simulink model "Bixler_w_autopilot_sepTaskRate"  (R2018b)
settings: Solver=FixedStepAuto  StartTime=0.0  StopTime=inf  RelTol=1e-3  EnableMultiTasking=on
undefined symbols (not defined in the file or in its folder): dev, Main, pwm_output0
libraries: simulink x5, px4uORBlib x5, aerolibutil x4, px4lib x2, px4Sensorslib x2, vrlib x1, sharedtransform x1
(part 1 of 2)
settings Model: xpc_rtwmakecfg_data=_xpcnblib_  SimulationMode=external  ExtModeTrigDuration=10  Creator=Robert  LastModifiedBy=Robert
settings SolverCC: PositivePriorityOrder=on
settings DataIOCC: SaveState=on
settings OptimizationCC: DefaultUnderspecifiedDataType=single  EnhancedBackFolding=on  PassReuseOutputArgsAs=Individual arguments  MaxStackSize=64  OptimizeBlockOrder=speed  DifferentSizesBufferReuse=on  OptimizationCustomize=off
settings DebuggingCC: ParameterTunabilityLossMsg=error
settings HardwareCC: ProdBitPerPointer=32  ProdBitPerSizeT=32  ProdBitPerPtrDiffT=32  ProdLargestAtomicInteger=Long  ProdLargestAtomicFloat=Double  ProdWordSize=32  ProdLongLongMode=on  ProdHWDeviceType=ARM Compatible->ARM Cortex
settings SFSimCC: MATLABDynamicMemAlloc=off
settings RTWCC: SystemTargetFile=ert.tlc  HardwareBoard=PX4 Pixhawk 1  TLCOptions="-aInlineSetEventsForThisBaseRateFcn=TLC_FALSE -aSuppressMultiTaskScheduler=TLC_FALSE  -aRateBasedStepFcn=0"  TemplateMakefile=ert_default_tmf  GenerateReport=on  Toolchain=GNU Tools for PX4 Autopilots  IncludeHyperlinkInReport=on  LaunchReport=on  TargetLang=C++  GenerateTraceInfo=on  GenerateTraceReport=on  GenerateTraceReportSl=on  GenerateTraceReportSf=on  GenerateTraceReportEml=on
settings CodeAppCC: ForceParamTrailComments=on  IgnoreCustomStorageClasses=off  OperatorAnnotations=on  SimulinkDataObjDesc=on  SFDataObjDesc=on  InsertBlockDesc=on
settings ERTTargetCC: ExtMode=on  ExtModeMexArgs='127.0.0.1' 1 17725

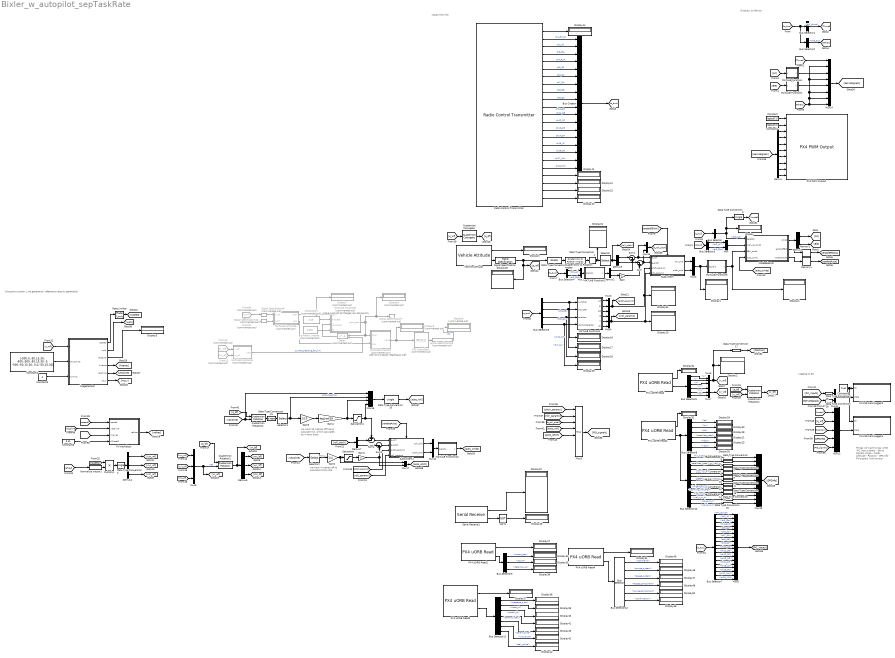
== system Bixler_w_autopilot_sepTaskRate ==
  note: Logging to SD
  note: Inputs from RC
  note: Outputs, to Servos
  note: Things we want to log:
      |
      | uint8
      | -RC input signals
      | - Servo Signals
      |
      | single
      | - Mode
      | - Attitude
      | - Position
      | - GPS info
      | - Pid signals (with errors)
  note: we want 4 metres off
      | to saturate climb rate
  note: Waypoint system,
      | Line generation,
      | reference velocity generation
  note: make sure not to change yaw too quickly
  note: Use roll to adjust heading as well
  note: we want 10 metres off
      | line to saturate roll, which
      | saturates as in next block
  Bus Creator : BusCreator  Inputs=18
  Bus Selector : BusSelector  OutputSignals=ch9_SC
  Bus Selector1 : BusSelector  OutputSignals=ch1_thrust
  Bus Selector10 : BusSelector  OutputSignals=fix_type,satellites_used,lat,lon,alt,hdop,vdop,noise_per_ms,jamming_indicator,vel_m_s,vel_n_m_s,vel_e_m_s,vel_d_m_s
  Bus Selector11 : BusSelector  OutputSignals=message_type,node_id,param_id,param_index,param_type,int_value,real_value
  Bus Selector12 : BusSelector  OutputSignals=command,source_system,target_system,target_component,source_component,confirmation
  Bus Selector2 : BusSelector  OutputSignals=ch6_S2
  Bus Selector3 : BusSelector  OutputSignals=ch2_Ail,ch3_Ele
  Bus Selector4 : BusSelector  OutputSignals=ch2_Ail,ch3_Ele
  Bus Selector5 : BusSelector  OutputSignals=ch8_SB,ch5_S1,ch12_SF,ch7_SA
  Bus Selector6 : BusSelector  OutputSignals=x,y,z,vx,vy,vz
  Bus Selector7 : BusSelector  OutputSignals=ch1_thrust,ch2_Ail,ch3_Ele,ch4_Rud,ch5_S1,ch6_S2,ch7_SA,ch8_SB,ch9_SC,ch10_SD,ch11_SE,ch12_SF,ch13_SG,ch14_SH,ch15_LS,ch16_RS,ch17_MAX,ch18_MIN
  Bus Selector8 : BusSelector  OutputSignals=lat,lon,alt,satellites_used,hdop,vdop
  Bus Selector9 : BusSelector  OutputSignals=current_seq,count,dataman_id
  Constant : Constant  Value=logical(1)
  Constant1 : Constant  Value=logical(0)
  Constant11 : Constant  Commented=on  Value=0.15  OutDataTypeStr=single  SampleTime=1/250
  Constant2 : Constant  Value=[-500,0,-50,15,30; -500,-500,-50,15,30; 0, -500,-50,15,30; 0,0,-50,15,30]  OutDataTypeStr=single
  Constant3 : Constant  Value=4  OutDataTypeStr=single
  Constant5 : Constant  Value=0.11  OutDataTypeStr=single  SampleTime=-1
  Constant8 : Constant  Value=true  OutDataTypeStr=boolean  SampleTime=0.004
  Data Type Conversion : DataTypeConversion  OutDataTypeStr=double
  Data Type Conversion{1..17,20..21} (19 alike) : DataTypeConversion  OutDataTypeStr=single
  Data Type Conversion18 : DataTypeConversion  OutDataTypeStr=uint16
  Data Type Conversion19 : DataTypeConversion  OutDataTypeStr=uint16
  Delay : Delay  Commented=on  DelayLength=1  InitialConditionSource=Input port
      settings: InputPortMap=u0,p4
  Demux : Demux  Outputs=8
  Demux{1..3,7} (4 alike) : Demux  Outputs=2
  Demux4 : Demux  Outputs=3
  Demux5 : Demux  Outputs=3
  Display{,1..5,10..51} (48 alike) : Display
  Display{6..9} (4 alike) : Display  Commented=on
  FlyVecAdjust : MATLAB Function  TreatAsAtomicUnit=on
  From12 : From  Commented=on  GotoTag=v_wf
  From13 : From  Commented=on  GotoTag=vr_wf
  From56 : From  Commented=on  GotoTag=vr_wf
  From57 : From  Commented=on  GotoTag=v_wf
  Gain : Gain  Gain=-1
  Gain1 : Gain  Gain=-1
  Gain2 : Gain  Gain=1/4
  Gain3 : Gain  Gain=1/10
  Gain4 : Gain  Gain=deg2rad(30)
  MATLAB Function : MATLAB Function  TreatAsAtomicUnit=on
  MATLAB Function1 : MATLAB Function  TreatAsAtomicUnit=on
  MATLAB Function10 : MATLAB Function  TreatAsAtomicUnit=on
  MATLAB Function2 : MATLAB Function  TreatAsAtomicUnit=on
  MATLAB Function3 : MATLAB Function  TreatAsAtomicUnit=on
  MATLAB Function4 : MATLAB Function  TreatAsAtomicUnit=on
  MATLAB Function5 : MATLAB Function  Commented=on  TreatAsAtomicUnit=on
  MATLAB Function6 : MATLAB Function  Commented=on  TreatAsAtomicUnit=on
  MATLAB Function7 : MATLAB Function  Commented=on  TreatAsAtomicUnit=on
  MATLAB Function8 : MATLAB Function  Commented=on  TreatAsAtomicUnit=on
  Memory1 : Memory  InheritSampleTime=on
  Memory2 : Memory  InheritSampleTime=on
  ModeSelector : MATLAB Function  TreatAsAtomicUnit=on
  Multiply1 : Product
  Mux{,1..2,10..11,15,17} (7 alike) : Mux  Inputs=2
  Mux12 : Mux  Inputs=5
  Mux13 : Mux  Inputs=13
  Mux14 : Mux  Inputs=8
  Mux16 : Mux
  Mux{3..7} (5 alike) : Mux  Inputs=3
  Mux8 : Mux  Inputs=18
  Mux9 : Mux  Inputs=8
  NOT1 : Logic  Operator=NOT  IconShape=distinctive  AllPortsSameDT=off  OutDataTypeStr=boolean
  Normalize Vector1 : vrlib/Utilities/Normalize Vector  maxzero=0
      settings: SourceProductName=Simulink 3D Animation  SourceProductBaseCode=VR
  PID Controller2 : simulink/Continuous/PID Controller  Commented=on  Controller=PID  Form=Parallel  TimeDomain=Discrete-time  SampleTime=-1  IntegratorMethod=Forward Euler  FilterMethod=Forward Euler  ControllerParametersSource=internal  P=1  I=0  D=0.5*0  UseFilter=off  N=100  TunerSelectOption=Transfer Function Based (PID Tuner App)  InitialConditionSource=internal  InitialConditionForIntegrator=0  InitialConditionForFilter=0  DifferentiatorICPrevScaledInput=0  ExternalReset=none  TrackingMode=off  Kt=1  LimitOutput=on  UpperSaturationLimit=deg2rad(30)  LowerSaturationLimit=-deg2rad(30)  LinearizeAsGain=on  AntiWindupMode=clamping  Kb=1  POutMin=[]  POutMax=[]  IOutMin=[]  IOutMax=[]  DOutMin=[]  DOutMax=[]  NOutMin=[]  NOutMax=[]  SumOutMin=[]  SumOutMax=[]  SaturationOutMin=[]  SaturationOutMax=[]  PParamMin=[]  PParamMax=[]  IParamMin=[]  IParamMax=[]  DParamMin=[]  DParamMax=[]  NParamMin=[]  NParamMax=[]  KbParamMin=[]  KbParamMax=[]  KtParamMin=[]  KtParamMax=[]  KbOutMin=[]  KbOutMax=[]  KtOutMin=[]  KtOutMax=[]  IntegratorOutMin=[]  IntegratorOutMax=[]  FilterOutMin=[]  FilterOutMax=[]  SumI1OutMin=[]  SumI1OutMax=[]  SumI2OutMin=[]  SumI2OutMax=[]  SumI3OutMin=[]  SumI3OutMax=[]  SumI4OutMin=[]  SumI4OutMax=[]  SumDOutMin=[]  SumDOutMax=[]  DifferentiatorOutMin=[]  DifferentiatorOutMax=[]  FilterDiffOutCoefMin=[]  FilterDiffOutCoefMax=[]  ReciprocalOutMin=[]  ReciprocalOutMax=[]  SumDenOutMin=[]  SumDenOutMax=[]  SumNumOutMin=[]  SumNumOutMax=[]  DivideOutMin=[]  DivideOutMax=[]  IntegratorContinuousStateAttributes=''  IntegratorStateMustResolveToSignalObject=off  IntegratorRTWStateStorageClass=Auto  FilterContinuousStateAttributes=''  FilterStateMustResolveToSignalObject=off  FilterRTWStateStorageClass=Auto  ParallelPVariant=InternalParameters  IdealPVariant=Disabled  IVariant=InternalParameters  DVariant=InternalParameters  IntegratorVariant=Discrete  SatVariant=Enabled  AWVariant=DiscClampingParallel  PCopyVariant=Disabled  TRVariant=Disabled  FdbkBlocksVariant=Forward  IdealPFdbkVariant=Disabled  SatFdbkVariant=Disabled  DerivativeFilterVariant=Differentiator  NVariant=Passthrough  NCopyVariant=Disabled_SignalSpec  FilterICVariant=InternalICsDifferentiator  IntegratorICVariant=InternalICs  ExternalResetVariant=Disabled  TRSumVariant=Passthrough  SumFdbkVariant=Disabled  SumVariant=Sum_PID
  PX4 PWM Output : px4lib/PX4 PWM Output  pwmDevice=Main (/dev/pwm_output0)  pwmChannel1_=on  pwmChannel2_=on  pwmChannel3_=on  pwmChannel4_=on  pwmChannel5_=on  pwmChannel6_=on  pwmChannel7_=on  pwmChannel8_=on  forceTerminateFailsafe=off  outputErrorStatus=off
      settings: SourceProductName=Embedded Coder Support Package for PX4 Autopilots
  PX4 SD Card Logger2 : Subsystem  mask(PX4 SD Card Logger){logfile=/fs/microsd/log, logfilename=rc_and_servosignals, cacheflag=off, numRecs=250*60*60}
      mask prompts: logfile "Log Folder"; logfilename "Log File Name"; cacheflag "Cache in Memory"; numRecs "Maximum Record Count"
      mask help:
      | Log data to a specified file on the SD card
      |
      | The block accepts two inputs, enable and data. The incoming data is logged into the SD card when the enable signal is high and the number of data points logged is less than the Maximum Record Count specified.
      |
      | The specified folder should be present in the SD card for logging.
      |
      | If Cache in Memory is unchecked, the data is written to the SD card at every timestep.  If Cache in Memory is checked, data is cached in the memory and is written to SD card only when enable goes low or when the number of data points logged reaches the Maximum Record Count specified.
      mask init:
      | logname=uint8([logfile,'/',logfilename]);
      mask Help: eval('codertarget.internal.helpView(''px4'',''px4sdcardexample'')');
      mask Display:
      | fprintf([get_param(gcb,'logfile'),'/',get_param(gcb,'logfilename')])
      | port_label('input',1,'en')
      | port_label('input',2,'data')
  PX4 SD Card Logger4 : Subsystem  mask(PX4 SD Card Logger){logfile=/fs/microsd/log, logfilename=MainLog, cacheflag=off, numRecs=250*60*60}
      mask prompts: logfile "Log Folder"; logfilename "Log File Name"; cacheflag "Cache in Memory"; numRecs "Maximum Record Count"
      mask help:
      | Log data to a specified file on the SD card
      |
      | The block accepts two inputs, enable and data. The incoming data is logged into the SD card when the enable signal is high and the number of data points logged is less than the Maximum Record Count specified.
      |
      | The specified folder should be present in the SD card for logging.
      |
      | If Cache in Memory is unchecked, the data is written to the SD card at every timestep.  If Cache in Memory is checked, data is cached in the memory and is written to SD card only when enable goes low or when the number of data points logged reaches the Maximum Record Count specified.
      mask init:
      | logname=uint8([logfile,'/',logfilename]);
      mask Help: eval('codertarget.internal.helpView(''px4'',''px4sdcardexample'')');
      mask Display:
      | fprintf([get_param(gcb,'logfile'),'/',get_param(gcb,'logfilename')])
      | port_label('input',1,'en')
      | port_label('input',2,'data')
  PX4 uORB Read : px4uORBlib/PX4 uORB Read  uORBTopic=vehicle_local_position  sampleTime=0.004  BlockingMode=off  BlockTimeout=1e-3
      settings: SourceProductName=Embedded Coder Support Package for PX4 Autopilots
  PX4 uORB Read1 : px4uORBlib/PX4 uORB Read  uORBTopic=mission  sampleTime=-1  BlockingMode=off  BlockTimeout=1e-3
      settings: SourceProductName=Embedded Coder Support Package for PX4 Autopilots
  PX4 uORB Read2 : px4uORBlib/PX4 uORB Read  uORBTopic=vehicle_gps_position  sampleTime=0.004  BlockingMode=off  BlockTimeout=1e-3
      settings: SourceProductName=Embedded Coder Support Package for PX4 Autopilots
  PX4 uORB Read3 : px4uORBlib/PX4 uORB Read  uORBTopic=uavcan_parameter_request  sampleTime=-1  BlockingMode=off  BlockTimeout=1e-3
      settings: SourceProductName=Embedded Coder Support Package for PX4 Autopilots
  PX4 uORB Read4 : px4uORBlib/PX4 uORB Read  uORBTopic=vehicle_command  sampleTime=-1  BlockingMode=off  BlockTimeout=1e-3
      settings: SourceProductName=Embedded Coder Support Package for PX4 Autopilots
  Quaternion Conjugate : aerolibutil/Quaternion Conjugate
      settings: SourceProductName=Aerospace Blockset  SourceProductBaseCode=AE
  Quaternion Rotation1 : aerolibutil/Quaternion Rotation
  Quaternion Rotation2 : aerolibutil/Quaternion Rotation
  Quaternion Rotation4 : aerolibutil/Quaternion Rotation
  Quaternions to Rotation Angles : sharedtransform/Quaternions to Rotation Angles  rotationOrder=ZYX  aMode=aMode
      settings: SourceProductBaseCode=AE
  Radio Control Transmitter : px4Sensorslib/Radio Control Transmitter  channel1=on  channel2=on  channel3=on  channel4=on  channel5=on  channel6=on  channel7=on  channel8=on  channel9=on  channel10=on  channel11=on  channel12=on  channel13=on  channel14=on  channel15=on  channel16=on  channel17=on  channel18=on  channel_count=on  rssi=on  rc_input_source=on  timestamp_last_signal=on  time_stamp=off  sampleTime=1/250  BlockingMode=off  BlockTimeout=5
      settings: SourceProductName=Embedded Coder Support Package for PX4 Autopilots
  Rate Limiter : RateLimiter  SampleTimeMode=inherited  InitialCondition=0.01
  Saturation : Saturate  UpperLimit=deg2rad(15)  LowerLimit=deg2rad(-20)
  Saturation1 : Saturate  UpperLimit=deg2rad(30)  LowerLimit=deg2rad(-30)
  Selector : Selector  InputPortWidth=3  IndexOptions=Index vector (dialog)  Indices=[3 2]  OutputSizes=1
  Selector1 : Selector  InputPortWidth=3  IndexOptions=Index vector (dialog)  Indices=[2]  OutputSizes=1
  Selector2 : Selector  InputPortWidth=3  IndexOptions=Index vector (dialog)  Indices=[3]  OutputSizes=1
  Serial Receive1 : px4lib/Serial Receive  SCIModule=/dev/ttyS2  DataType=uint8  DataLength=10  OutputStatus=on  SampleTime=-1  BlockingMode=off  PartialData=on  Timeout=5
      settings: SourceProductName=Embedded Coder Support Package for PX4 Autopilots  SourceProductBaseCode=PX4AUTOPILOTS
  Signal Specification : SignalSpecification  OutDataTypeStr=single
  Signal Specification10 : SignalSpecification  Commented=on  OutDataTypeStr=single  Dimensions=3
  Signal Specification7 : SignalSpecification  Commented=on  OutDataTypeStr=single  Dimensions=1
  Signal Specification8 : SignalSpecification  Commented=on  OutDataTypeStr=single  Dimensions=1
  Signal Specification9 : SignalSpecification  Commented=on  OutDataTypeStr=single  Dimensions=3
  Subsystem : Subsystem
  Subsystem1 : Subsystem
  Sum : Sum  Inputs=|-+
  Sum1 : Sum  Inputs=|-+
  Sum3 : Sum  Inputs=|-+
  Sum4 : Sum  Inputs=+-|
  Vehicle Attitude : px4Sensorslib/Vehicle Attitude  rollRate=off  pitchRate=off  yawRate=off  quaternion=on  uorbTimeStamp=off  BlockingMode=off  BlockTimeout=0.001  sampleTime=1/250
      settings: SourceProductName=Embedded Coder Support Package for PX4 Autopilots
  linegenerator : MATLAB Function  TreatAsAtomicUnit=on
  "pixhawk_maybe " : Constant  Commented=on  Value=0.004  OutDataTypeStr=single  SampleTime=1/250
  wires:
  Vehicle Attitude/2 -> Signal Specification/1
  Vehicle Attitude/1 -> Display3/1
  Radio Control Transmitter/8 -> Bus Creator/7  "ch7_SA"
  Radio Control Transmitter/7 -> Bus Creator/6  "ch6_S2"
  Radio Control Transmitter/6 -> Bus Creator/5  "ch5_S1"
  Radio Control Transmitter/2 -> Bus Creator/1  "ch1_thrust"
  Radio Control Transmitter/3 -> Bus Creator/2  "ch2_Ail"
  Radio Control Transmitter/4 -> Bus Creator/3  "ch3_Ele"
  Radio Control Transmitter/5 -> Bus Creator/4  "ch4_Rud"
  Radio Control Transmitter/9 -> Bus Creator/8  "ch8_SB"
  Radio Control Transmitter/20 -> Display11/1
  Radio Control Transmitter/21 -> Display12/1
  Radio Control Transmitter/23 -> Display13/1
  Radio Control Transmitter/1 -> Display14/1
  Radio Control Transmitter/22 -> Display15/1
  Constant/1 -> PX4 PWM Output/1
  Bus Selector1/1 -> [Thrust]  "<ch1_thrust>"
  [Others] -> Mux14/8, Mux14/7, Mux14/6, Mux14/4, Mux14/2
  Constant1/1 -> PX4 PWM Output/2
  Bus Creator/1 -> [rc_bus]
  Quaternions to Rotation Angles/1 -> Data Type Conversion1/1
  Bus Selector/1 -> ModeSelector/1(selector), Display/1, Data Type Conversion3/1  "<ch9_SC>"
  Demux3/1 -> Sum1/1
  Demux3/2 -> Sum/1
  Mux2/1 -> Display1/1, MATLAB Function3/1(signals)
  Signal Specification/1 -> [q_wf], Display25/1, Data Type Conversion/1
  [rc_bus] -> Bus Selector2/1, Bus Selector1/1
  [Thrust] -> Mux14/1
  [Ail] -> MATLAB Function/1(u)
  [Ele] -> MATLAB Function1/1(u)
  [rc_bus] -> Bus Selector3/1
  [rc_bus] -> Bus Selector/1
  MATLAB Function3/1(y) -> ModeSelector/3(FBW_cmds), Display4/1
  Bus Selector3/1 -> Mux/1  "<ch2_Ail>"
  Bus Selector3/2 -> Mux/2  "<ch3_Ele>"
  Mux/1 -> ModeSelector/2(manual_cmds)
  ModeSelector/1(cmds) -> Demux1/1
  Demux1/1 -> [Ail]
  Demux1/2 -> [Ele]
  Bus Selector2/1 -> [Others]  "<ch6_S2>"
  Data Type Conversion/1 -> Quaternions to Rotation Angles/1
  MATLAB Function/1(y) -> Mux14/3
  MATLAB Function1/1(y) -> Mux14/5
  Demux2/2 -> Gain/1
  [rc_bus] -> Bus Selector4/1
  Bus Selector4/1 -> Mux1/1  "<ch2_Ail>"
  Bus Selector4/2 -> Mux1/2  "<ch3_Ele>"
  Mux1/1 -> MATLAB Function2/1(signals)
  MATLAB Function2/1(y) -> Demux2/1
  Demux2/1 -> Sum1/2
  Mux4/1 -> [roll_params], Subsystem/4(roll_params), Display10/1
  [rc_bus] -> Bus Selector5/1
  Bus Selector5/2 -> Display17/1, MATLAB Function4/2(adjuster)  "<ch5_S1>"
  Bus Selector5/1 -> Display16/1, MATLAB Function4/1(switcher)  "<ch8_SB>"
  MATLAB Function4/1(pP) -> Mux3/1
  MATLAB Function4/2(pI) -> Mux3/2
  MATLAB Function4/3(pD) -> Mux3/3
  Bus Selector5/3 -> Display18/1, MATLAB Function4/3(enabler)  "<ch12_SF>"
  Radio Control Transmitter/10 -> Bus Creator/9  "ch9_SC"
  Radio Control Transmitter/11 -> Bus Creator/10  "ch10_SD"
  Radio Control Transmitter/12 -> Bus Creator/11  "ch11_SE"
  Radio Control Transmitter/13 -> Bus Creator/12  "ch12_SF"
  Radio Control Transmitter/14 -> Bus Creator/13  "ch13_SG"
  Radio Control Transmitter/15 -> Bus Creator/14  "ch14_SH"
  Radio Control Transmitter/16 -> Bus Creator/15  "ch15_LS"
  Radio Control Transmitter/17 -> Bus Creator/16  "ch16_RS"
  Radio Control Transmitter/18 -> Bus Creator/17  "ch17_MAX"
  Radio Control Transmitter/19 -> Bus Creator/18  "ch18_MIN"
  MATLAB Function4/4(rP) -> Mux4/1
  MATLAB Function4/5(rI) -> Mux4/2
  MATLAB Function4/6(rD) -> Mux4/3
  Bus Selector5/4 -> Display19/1, MATLAB Function4/4(ControlSelector)  "<ch7_SA>"
  PX4 uORB Read/2 -> Bus Selector6/1
  PX4 uORB Read2/2 -> Bus Selector10/1, Bus Selector8/1
  PX4 uORB Read/1 -> Display34/1
  PX4 uORB Read2/1 -> Display32/1
  Bus Selector6/1 -> Mux5/1  "<x>"
  Bus Selector6/2 -> Mux5/2  "<y>"
  Bus Selector6/3 -> Mux5/3  "<z>"
  Bus Selector8/1 -> Display29/1  "<lat>"
  Bus Selector8/2 -> Display30/1  "<lon>"
  Bus Selector8/3 -> Display28/1  "<alt>"
  Sum1/1 -> Mux15/1, Subsystem/1(e_roll)
  Sum/1 -> Subsystem/2(e_pitch), Mux15/2
  Subsystem/1(roll_cmd) -> Mux2/1
  Subsystem/2(pitch_cmd) -> Mux2/2
  [enableFBWA] -> Subsystem/Enable
  Gain/1 -> Sum/2
  Mux3/1 -> [pitch_params], Subsystem/3(pitch_params), Display31/1
  ModeSelector/2(enableFBW) -> Memory2/1
  Selector/1 -> [roll_pitch], Demux3/1
  ModeSelector/3(enableAuto) -> Memory1/1
  Memory1/1 -> [enableAuto]
  Memory2/1 -> [enableFBWA]
  Mux5/1 -> Data Type Conversion17/1, Display2/1, [r_wf]
  [rspeed] -> Multiply1/1
  linegenerator/1(rspeed) -> Rate Limiter/1
  linegenerator/2(wpN) -> [wpN]
  linegenerator/4(linevec) -> [linevec]
  Constant5/1 -> FlyVecAdjust/4(d2lcoeff)
  [linevec] -> FlyVecAdjust/3(linevec)
  [refvec] -> Normalize Vector1/1
  [vec2line] -> FlyVecAdjust/2(vec2line)
  Normalize Vector1/1 -> Multiply1/2
  linegenerator/6(wp_r) -> [wp_r]
  Rate Limiter/1 -> [rspeed]
  Demux4/1 -> [vxr_wf]
  FlyVecAdjust/1(refvec) -> [refvec]
  Demux4/2 -> [vyr_wf]
  Demux4/3 -> [vzr_wf]
  linegenerator/5(vec2line) -> [vec2line]
  [rspeed] -> FlyVecAdjust/1(rspeed)
  Multiply1/1 -> Data Type Conversion2/1
  From12/1 -> MATLAB Function5/1(v_wf)
  From13/1 -> MATLAB Function5/2(vr_wf)
  [r_wf] -> linegenerator/1(r)
  linegenerator/3(dist2wp) -> Display5/1
  [vzr_wf] -> Mux6/3
  [vyr_wf] -> Mux6/2
  [vxr_wf] -> Mux6/1
  Demux5/2 -> [vyr_bf]
  Demux5/3 -> [vzr_bf]
  Demux5/1 -> [vxr_bf]
  Quaternion Rotation1/1 -> Demux5/1, [vr_bf]
  [q_bf] -> Quaternion Rotation1/1
  Mux6/1 -> [vr_wf], Quaternion Rotation1/2  "vref"
  [q_wf] -> Quaternion Conjugate/1
  Quaternion Conjugate/1 -> [q_bf]
  Bus Selector6/4 -> Mux7/1  "<vx>"
  Bus Selector6/5 -> Mux7/2  "<vy>"
  Bus Selector6/6 -> Mux7/3  "<vz>"
  Mux7/1 -> [v_wf]
  Quaternion Rotation4/1 -> [v_bf]
  [v_wf] -> Quaternion Rotation4/2
  [q_bf] -> Quaternion Rotation4/1
  [auto_cmds] -> ModeSelector/4(auto_cmds)
  MATLAB Function5/1(yaw) -> Delay/2  "currrent_heading_for_init"
  From56/1 -> Signal Specification9/1
  PID Controller2/1 -> Signal Specification8/1
  Delay/1 -> MATLAB Function6/3(yawr_last)
  From57/1 -> Signal Specification10/1
  MATLAB Function8/2(yaw) -> MATLAB Function7/2(yaw)
  Signal Specification9/1 -> MATLAB Function8/1(vr_wf)
  MATLAB Function8/1(yawr) -> Display7/1, MATLAB Function6/1(yawr)
  Signal Specification8/1 -> Display6/1  "roll"
  MATLAB Function7/1(yawe) -> Display9/1, PID Controller2/1
  Signal Specification10/1 -> MATLAB Function8/2(v_wf)
  Constant11/1 -> MATLAB Function6/2(maxrate)
  MATLAB Function6/1(yawr_slow) -> Display8/1, Signal Specification7/1, Delay/1, MATLAB Function7/1(yawr)
  [vec2line] -> Selector2/1
  Selector2/1 -> Gain2/1  "error_z"
  Subsystem1/1(roll_cmd) -> Mux10/1
  Gain1/1 -> Sum3/2, Mux17/2
  Subsystem1/2(pitch_cmd) -> Mux10/2
  Sum4/1 -> Subsystem1/1(e_roll)
  Sum3/1 -> Subsystem1/2(e_pitch)
  [enableAuto] -> Subsystem1/Enable
  Gain2/1 -> Mux17/1, Saturation/1
  Demux7/2 -> Sum3/1
  Demux7/1 -> Sum4/2
  [pitch_params] -> Subsystem1/3(pitch_params)
  [roll_params] -> Subsystem1/4(roll_params)
  [roll_pitch] -> Demux7/1
  Mux10/1 -> MATLAB Function10/1(signals)
  MATLAB Function10/1(y) -> [auto_cmds]
  "pixhawk_maybe "/1 -> MATLAB Function6/4(Ts)
  Constant2/1 -> linegenerator/2(waypoints)
  Constant3/1 -> linegenerator/3(numwp)
  Data Type Conversion2/1 -> Demux4/1
  Saturation/1 -> Gain1/1
  Bus Selector8/4 -> Display21/1  "<satellites_used>"
  Bus Selector8/5 -> Display23/1  "<hdop>"
  Bus Selector8/6 -> Display20/1  "<vdop>"
  Data Type Conversion1/1 -> Display24/1, Selector/1
  Constant8/1 -> PX4 SD Card Logger4/1(En), PX4 SD Card Logger2/1(En)
  Mux11/1 -> PX4 SD Card Logger2/2(Data)
  [RC_inputs] -> Data Type Conversion18/1
  [ServoSignals] -> Data Type Conversion19/1
  Mux12/1 -> PX4 SD Card Logger4/2(Data)
  [mode] -> Mux12/1
  [q_wf] -> Mux12/2
  [Position] -> Mux12/3
  [GPSinfo] -> Mux12/4
  [PID_signals] -> Mux12/5
  Bus Selector10/1 -> Data Type Conversion4/1  "<fix_type>"
  Bus Selector10/2 -> Data Type Conversion5/1  "<satellites_used>"
  Bus Selector10/3 -> Data Type Conversion6/1  "<lat>"
  Bus Selector10/4 -> Data Type Conversion7/1  "<lon>"
  Bus Selector10/5 -> Data Type Conversion8/1  "<alt>"
  Bus Selector10/6 -> Data Type Conversion9/1  "<hdop>"
  Bus Selector10/7 -> Data Type Conversion10/1  "<vdop>"
  Bus Selector10/8 -> Data Type Conversion11/1  "<noise_per_ms>"
  Bus Selector10/9 -> Data Type Conversion12/1  "<jamming_indicator>"
  Bus Selector10/10 -> Data Type Conversion13/1  "<vel_m_s>"
  Bus Selector10/11 -> Data Type Conversion14/1  "<vel_n_m_s>"
  Bus Selector10/12 -> Data Type Conversion15/1  "<vel_e_m_s>"
  Bus Selector10/13 -> Data Type Conversion16/1  "<vel_d_m_s>"
  Mux13/1 -> [GPSinfo]
  Data Type Conversion3/1 -> [mode]
  [rc_bus] -> Bus Selector7/1
  Bus Selector7/1 -> Mux8/1  "<ch1_thrust>"
  Bus Selector7/2 -> Mux8/2  "<ch2_Ail>"
  Bus Selector7/3 -> Mux8/3  "<ch3_Ele>"
  Bus Selector7/4 -> Mux8/4  "<ch4_Rud>"
  Bus Selector7/5 -> Mux8/5  "<ch5_S1>"
  Bus Selector7/6 -> Mux8/6  "<ch6_S2>"
  Bus Selector7/7 -> Mux8/7  "<ch7_SA>"
  Bus Selector7/8 -> Mux8/8  "<ch8_SB>"
  Bus Selector7/9 -> Mux8/9  "<ch9_SC>"
  Bus Selector7/10 -> Mux8/10  "<ch10_SD>"
  Bus Selector7/11 -> Mux8/11  "<ch11_SE>"
  Bus Selector7/12 -> Mux8/12  "<ch12_SF>"
  Bus Selector7/13 -> Mux8/13  "<ch13_SG>"
  Bus Selector7/14 -> Mux8/14  "<ch14_SH>"
  Bus Selector7/15 -> Mux8/15  "<ch15_LS>"
  Bus Selector7/16 -> Mux8/16  "<ch16_RS>"
  Bus Selector7/17 -> Mux8/17  "<ch17_MAX>"
  Bus Selector7/18 -> Mux8/18  "<ch18_MIN>"
  Mux8/1 -> [RC_inputs]
  Mux14/1 -> [ServoSignals]
  Demux/1 -> PX4 PWM Output/3
  Demux/2 -> PX4 PWM Output/4
  Demux/3 -> PX4 PWM Output/5
  Demux/4 -> PX4 PWM Output/6
  Demux/5 -> PX4 PWM Output/7
  Demux/6 -> PX4 PWM Output/8
  Demux/7 -> PX4 PWM Output/9
  Demux/8 -> PX4 PWM Output/10
  [ServoSignals] -> Demux/1
  Mux9/1 -> [PID_signals]
  [pitch_params] -> Mux9/1
  [roll_params] -> Mux9/2
  Mux15/1 -> [e_roll_pitch]
  [e_roll_pitch] -> Mux9/3
  [vec2line] -> Mux16/1, Quaternion Rotation2/2
  [q_bf] -> Quaternion Rotation2/1
  Quaternion Rotation2/1 -> Data Type Conversion21/1
  Selector1/1 -> Mux16/2, Gain3/1  "error_heading"
  Gain3/1 -> Gain4/1
  Saturation1/1 -> Mux16/4, Sum4/1
  Gain4/1 -> Mux16/3, Saturation1/1
  Data Type Conversion4/1 -> Mux13/1
  Data Type Conversion5/1 -> Mux13/2
  Data Type Conversion6/1 -> Mux13/3
  Data Type Conversion7/1 -> Mux13/4
  Data Type Conversion8/1 -> Mux13/5
  Data Type Conversion9/1 -> Mux13/6
  Data Type Conversion10/1 -> Mux13/7
  Data Type Conversion11/1 -> Mux13/8
  Data Type Conversion12/1 -> Mux13/9
  Data Type Conversion13/1 -> Mux13/10
  Data Type Conversion14/1 -> Mux13/11
  Data Type Conversion15/1 -> Mux13/12
  Data Type Conversion16/1 -> Mux13/13
  Data Type Conversion17/1 -> [Position]
  Data Type Conversion18/1 -> Mux11/1
  Data Type Conversion19/1 -> Mux11/2
  Mux16/1 -> Data Type Conversion20/1
  Data Type Conversion20/1 -> [auto_roll]
  [auto_roll] -> Mux9/4
  Mux17/1 -> [auto_pitch]
  [auto_pitch] -> Mux9/5
  Data Type Conversion21/1 -> Selector1/1
  Serial Receive1/1 -> Display22/1
  Serial Receive1/2 -> NOT1/1
  NOT1/1 -> Display26/1
  PX4 uORB Read1/2 -> Bus Selector9/1
  PX4 uORB Read1/1 -> Display27/1
  Bus Selector9/2 -> Display35/1  "<count>"
  Bus Selector9/1 -> Display33/1  "<current_seq>"
  Bus Selector9/3 -> Display36/1  "<dataman_id>"
  PX4 uORB Read3/2 -> Bus Selector11/1
  PX4 uORB Read3/1 -> Display37/1
  Bus Selector11/1 -> Display38/1  "<message_type>"
  Bus Selector11/2 -> Display39/1  "<node_id>"
  Bus Selector11/3 -> Display40/1  "<param_id>"
  Bus Selector11/4 -> Display41/1  "<param_index>"
  Bus Selector11/5 -> Display43/1  "<param_type>"
  Bus Selector11/6 -> Display42/1  "<int_value>"
  Bus Selector11/7 -> Display44/1  "<real_value>"
  PX4 uORB Read4/2 -> Bus Selector12/1
  Bus Selector12/1 -> Display45/1  "<command>"
  Bus Selector12/2 -> Display46/1  "<source_system>"
  Bus Selector12/3 -> Display47/1  "<target_system>"
  Bus Selector12/4 -> Display48/1  "<target_component>"
  Bus Selector12/5 -> Display50/1  "<source_component>"
  Bus Selector12/6 -> Display49/1  "<confirmation>"
  PX4 uORB Read4/1 -> Display51/1

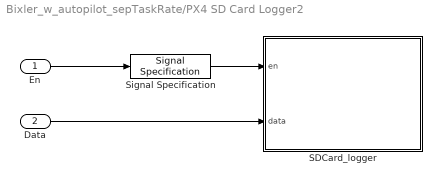
== system Bixler_w_autopilot_sepTaskRate/PX4 SD Card Logger2 ==
  En : Inport
  Data : Inport  Port=2
  SDCard_logger : MATLAB Function  TreatAsAtomicUnit=on
  Signal Specification : SignalSpecification  OutDataTypeStr=boolean
  wires:
  Signal Specification/1 -> SDCard_logger/1(en)
  En/1 -> Signal Specification/1
  Data/1 -> SDCard_logger/2(data)

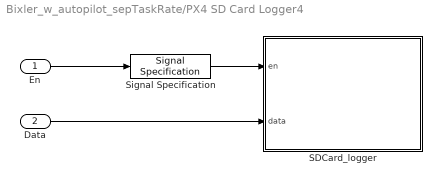
== system Bixler_w_autopilot_sepTaskRate/PX4 SD Card Logger4 ==
  En : Inport
  Data : Inport  Port=2
  SDCard_logger : MATLAB Function  TreatAsAtomicUnit=on
  Signal Specification : SignalSpecification  OutDataTypeStr=boolean
  wires:
  Signal Specification/1 -> SDCard_logger/1(en)
  En/1 -> Signal Specification/1
  Data/1 -> SDCard_logger/2(data)

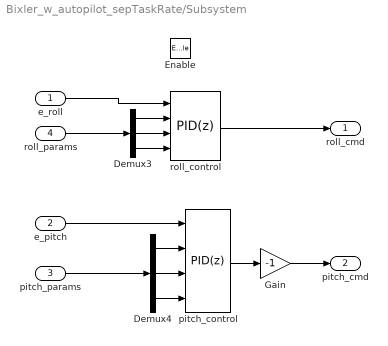
== system Bixler_w_autopilot_sepTaskRate/Subsystem ==
  e_roll : Inport
  e_pitch : Inport  Port=2
  pitch_params : Inport  Port=3
  roll_params : Inport  Port=4
  Enable : EnablePort
  Demux3 : Demux  Outputs=3
  Demux4 : Demux  Outputs=3
  Gain : Gain  Gain=-1
  pitch_control : simulink/Continuous/PID Controller  Controller=PID  Form=Parallel  TimeDomain=Discrete-time  SampleTime=1/250  IntegratorMethod=Backward Euler  FilterMethod=Forward Euler  ControllerParametersSource=external  P=1  I=0  D=0  UseFilter=off  N=100  TunerSelectOption=Transfer Function Based (PID Tuner App)  InitialConditionSource=internal  InitialConditionForIntegrator=0  InitialConditionForFilter=0  DifferentiatorICPrevScaledInput=0  ExternalReset=none  TrackingMode=off  Kt=1  LimitOutput=on  UpperSaturationLimit=1  LowerSaturationLimit=-1  LinearizeAsGain=off  AntiWindupMode=clamping  Kb=1  PGainOutDataTypeStr=single  PProdOutDataTypeStr=single  POutMin=[]  POutMax=[]  IGainOutDataTypeStr=single  IProdOutDataTypeStr=single  IOutMin=[]  IOutMax=[]  DGainOutDataTypeStr=single  DProdOutDataTypeStr=single  DOutMin=[]  DOutMax=[]  NOutMin=[]  NOutMax=[]  SumOutDataTypeStr=single  SumOutMin=[]  SumOutMax=[]  SaturationOutDataTypeStr=single  SaturationOutMin=[]  SaturationOutMax=[]  PParamDataTypeStr=single  PParamMin=[]  PParamMax=[]  IParamDataTypeStr=single  IParamMin=[]  IParamMax=[]  DParamDataTypeStr=single  DParamMin=[]  DParamMax=[]  NParamMin=[]  NParamMax=[]  KbParamMin=[]  KbParamMax=[]  KtParamMin=[]  KtParamMax=[]  KbOutMin=[]  KbOutMax=[]  KtOutMin=[]  KtOutMax=[]  IntegratorOutDataTypeStr=single  IntegratorOutMin=[]  IntegratorOutMax=[]  FilterOutMin=[]  FilterOutMax=[]  SumI1OutMin=[]  SumI1OutMax=[]  SumI2OutMin=[]  SumI2OutMax=[]  SumI3OutMin=[]  SumI3OutMax=[]  SumI4OutMin=[]  SumI4OutMax=[]  SumDOutMin=[]  SumDOutMax=[]  SumAccumDataTypeStr=single  DifferentiatorOutDataTypeStr=single  DifferentiatorOutMin=[]  DifferentiatorOutMax=[]  FilterDiffOutCoefMin=[]  FilterDiffOutCoefMax=[]  ReciprocalOutMin=[]  ReciprocalOutMax=[]  SumDenOutMin=[]  SumDenOutMax=[]  SumNumOutMin=[]  SumNumOutMax=[]  DivideOutMin=[]  DivideOutMax=[]  IntegratorContinuousStateAttributes=''  IntegratorStateMustResolveToSignalObject=off  IntegratorRTWStateStorageClass=Auto  FilterContinuousStateAttributes=''  FilterStateMustResolveToSignalObject=off  FilterRTWStateStorageClass=Auto  ParallelPVariant=ExternalParameters  IdealPVariant=Disabled  IVariant=ExternalParameters  DVariant=ExternalParameters  IntegratorVariant=Discrete  SatVariant=Enabled  AWVariant=DiscClampingParallel  PCopyVariant=Disabled  TRVariant=Disabled  FdbkBlocksVariant=Feedback  IdealPFdbkVariant=Passthrough  SatFdbkVariant=Passthrough  DerivativeFilterVariant=Differentiator  NVariant=Passthrough  NCopyVariant=Disabled_SignalSpec  FilterICVariant=InternalICsDifferentiator  IntegratorICVariant=InternalICs  ExternalResetVariant=Disabled  TRSumVariant=Passthrough  SumFdbkVariant=Enabled  SumVariant=Sum_PID
  roll_control : simulink/Continuous/PID Controller  Controller=PID  Form=Parallel  TimeDomain=Discrete-time  SampleTime=1/250  IntegratorMethod=Backward Euler  FilterMethod=Forward Euler  ControllerParametersSource=external  P=1  I=0  D=0  UseFilter=off  N=100  TunerSelectOption=Transfer Function Based (PID Tuner App)  InitialConditionSource=internal  InitialConditionForIntegrator=0  InitialConditionForFilter=0  DifferentiatorICPrevScaledInput=0  ExternalReset=none  TrackingMode=off  Kt=1  LimitOutput=on  UpperSaturationLimit=1  LowerSaturationLimit=-1  LinearizeAsGain=off  AntiWindupMode=clamping  Kb=1  PGainOutDataTypeStr=single  PProdOutDataTypeStr=single  POutMin=[]  POutMax=[]  IGainOutDataTypeStr=single  IProdOutDataTypeStr=single  IOutMin=[]  IOutMax=[]  DGainOutDataTypeStr=single  DProdOutDataTypeStr=single  DOutMin=[]  DOutMax=[]  NOutMin=[]  NOutMax=[]  SumOutDataTypeStr=single  SumOutMin=[]  SumOutMax=[]  SaturationOutDataTypeStr=single  SaturationOutMin=[]  SaturationOutMax=[]  PParamDataTypeStr=single  PParamMin=[]  PParamMax=[]  IParamDataTypeStr=single  IParamMin=[]  IParamMax=[]  DParamDataTypeStr=single  DParamMin=[]  DParamMax=[]  NParamMin=[]  NParamMax=[]  KbParamMin=[]  KbParamMax=[]  KtParamMin=[]  KtParamMax=[]  KbOutMin=[]  KbOutMax=[]  KtOutMin=[]  KtOutMax=[]  IntegratorOutDataTypeStr=single  IntegratorOutMin=[]  IntegratorOutMax=[]  FilterOutMin=[]  FilterOutMax=[]  SumI1OutMin=[]  SumI1OutMax=[]  SumI2OutMin=[]  SumI2OutMax=[]  SumI3OutMin=[]  SumI3OutMax=[]  SumI4OutMin=[]  SumI4OutMax=[]  SumDOutMin=[]  SumDOutMax=[]  SumAccumDataTypeStr=single  DifferentiatorOutDataTypeStr=single  DifferentiatorOutMin=[]  DifferentiatorOutMax=[]  FilterDiffOutCoefMin=[]  FilterDiffOutCoefMax=[]  ReciprocalOutMin=[]  ReciprocalOutMax=[]  SumDenOutMin=[]  SumDenOutMax=[]  SumNumOutMin=[]  SumNumOutMax=[]  DivideOutMin=[]  DivideOutMax=[]  IntegratorContinuousStateAttributes=''  IntegratorStateMustResolveToSignalObject=off  IntegratorRTWStateStorageClass=Auto  FilterContinuousStateAttributes=''  FilterStateMustResolveToSignalObject=off  FilterRTWStateStorageClass=Auto  ParallelPVariant=ExternalParameters  IdealPVariant=Disabled  IVariant=ExternalParameters  DVariant=ExternalParameters  IntegratorVariant=Discrete  SatVariant=Enabled  AWVariant=DiscClampingParallel  PCopyVariant=Disabled  TRVariant=Disabled  FdbkBlocksVariant=Feedback  IdealPFdbkVariant=Passthrough  SatFdbkVariant=Passthrough  DerivativeFilterVariant=Differentiator  NVariant=Passthrough  NCopyVariant=Disabled_SignalSpec  FilterICVariant=InternalICsDifferentiator  IntegratorICVariant=InternalICs  ExternalResetVariant=Disabled  TRSumVariant=Passthrough  SumFdbkVariant=Enabled  SumVariant=Sum_PID
  roll_cmd : Outport
  pitch_cmd : Outport  Port=2
  wires:
  roll_control/1 -> roll_cmd/1
  Demux4/3 -> pitch_control/4
  Demux4/2 -> pitch_control/3
  Demux4/1 -> pitch_control/2
  pitch_params/1 -> Demux4/1
  Demux3/3 -> roll_control/4
  Demux3/2 -> roll_control/3
  Demux3/1 -> roll_control/2
  pitch_control/1 -> Gain/1
  e_roll/1 -> roll_control/1
  e_pitch/1 -> pitch_control/1
  roll_params/1 -> Demux3/1
  Gain/1 -> pitch_cmd/1

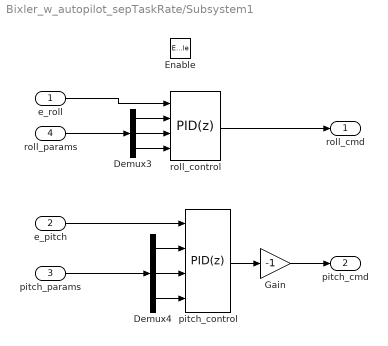
== system Bixler_w_autopilot_sepTaskRate/Subsystem1 ==
  e_roll : Inport
  e_pitch : Inport  Port=2
  pitch_params : Inport  Port=3
  roll_params : Inport  Port=4
  Enable : EnablePort
  Demux3 : Demux  Outputs=3
  Demux4 : Demux  Outputs=3
  Gain : Gain  Gain=-1
  pitch_control : simulink/Continuous/PID Controller  Controller=PID  Form=Parallel  TimeDomain=Discrete-time  SampleTime=1/250  IntegratorMethod=Backward Euler  FilterMethod=Forward Euler  ControllerParametersSource=external  P=1  I=0  D=0  UseFilter=off  N=100  TunerSelectOption=Transfer Function Based (PID Tuner App)  InitialConditionSource=internal  InitialConditionForIntegrator=0  InitialConditionForFilter=0  DifferentiatorICPrevScaledInput=0  ExternalReset=none  TrackingMode=off  Kt=1  LimitOutput=on  UpperSaturationLimit=1  LowerSaturationLimit=-1  LinearizeAsGain=off  AntiWindupMode=clamping  Kb=1  PGainOutDataTypeStr=single  PProdOutDataTypeStr=single  POutMin=[]  POutMax=[]  IGainOutDataTypeStr=single  IProdOutDataTypeStr=single  IOutMin=[]  IOutMax=[]  DGainOutDataTypeStr=single  DProdOutDataTypeStr=single  DOutMin=[]  DOutMax=[]  NOutMin=[]  NOutMax=[]  SumOutDataTypeStr=single  SumOutMin=[]  SumOutMax=[]  SaturationOutDataTypeStr=single  SaturationOutMin=[]  SaturationOutMax=[]  PParamDataTypeStr=single  PParamMin=[]  PParamMax=[]  IParamDataTypeStr=single  IParamMin=[]  IParamMax=[]  DParamDataTypeStr=single  DParamMin=[]  DParamMax=[]  NParamMin=[]  NParamMax=[]  KbParamMin=[]  KbParamMax=[]  KtParamMin=[]  KtParamMax=[]  KbOutMin=[]  KbOutMax=[]  KtOutMin=[]  KtOutMax=[]  IntegratorOutDataTypeStr=single  IntegratorOutMin=[]  IntegratorOutMax=[]  FilterOutMin=[]  FilterOutMax=[]  SumI1OutMin=[]  SumI1OutMax=[]  SumI2OutMin=[]  SumI2OutMax=[]  SumI3OutMin=[]  SumI3OutMax=[]  SumI4OutMin=[]  SumI4OutMax=[]  SumDOutMin=[]  SumDOutMax=[]  SumAccumDataTypeStr=single  DifferentiatorOutDataTypeStr=single  DifferentiatorOutMin=[]  DifferentiatorOutMax=[]  FilterDiffOutCoefMin=[]  FilterDiffOutCoefMax=[]  ReciprocalOutMin=[]  ReciprocalOutMax=[]  SumDenOutMin=[]  SumDenOutMax=[]  SumNumOutMin=[]  SumNumOutMax=[]  DivideOutMin=[]  DivideOutMax=[]  IntegratorContinuousStateAttributes=''  IntegratorStateMustResolveToSignalObject=off  IntegratorRTWStateStorageClass=Auto  FilterContinuousStateAttributes=''  FilterStateMustResolveToSignalObject=off  FilterRTWStateStorageClass=Auto  ParallelPVariant=ExternalParameters  IdealPVariant=Disabled  IVariant=ExternalParameters  DVariant=ExternalParameters  IntegratorVariant=Discrete  SatVariant=Enabled  AWVariant=DiscClampingParallel  PCopyVariant=Disabled  TRVariant=Disabled  FdbkBlocksVariant=Feedback  IdealPFdbkVariant=Passthrough  SatFdbkVariant=Passthrough  DerivativeFilterVariant=Differentiator  NVariant=Passthrough  NCopyVariant=Disabled_SignalSpec  FilterICVariant=InternalICsDifferentiator  IntegratorICVariant=InternalICs  ExternalResetVariant=Disabled  TRSumVariant=Passthrough  SumFdbkVariant=Enabled  SumVariant=Sum_PID
  roll_control : simulink/Continuous/PID Controller  Controller=PID  Form=Parallel  TimeDomain=Discrete-time  SampleTime=1/250  IntegratorMethod=Backward Euler  FilterMethod=Forward Euler  ControllerParametersSource=external  P=1  I=0  D=0  UseFilter=off  N=100  TunerSelectOption=Transfer Function Based (PID Tuner App)  InitialConditionSource=internal  InitialConditionForIntegrator=0  InitialConditionForFilter=0  DifferentiatorICPrevScaledInput=0  ExternalReset=none  TrackingMode=off  Kt=1  LimitOutput=on  UpperSaturationLimit=1  LowerSaturationLimit=-1  LinearizeAsGain=off  AntiWindupMode=clamping  Kb=1  PGainOutDataTypeStr=single  PProdOutDataTypeStr=single  POutMin=[]  POutMax=[]  IGainOutDataTypeStr=single  IProdOutDataTypeStr=single  IOutMin=[]  IOutMax=[]  DGainOutDataTypeStr=single  DProdOutDataTypeStr=single  DOutMin=[]  DOutMax=[]  NOutMin=[]  NOutMax=[]  SumOutDataTypeStr=single  SumOutMin=[]  SumOutMax=[]  SaturationOutDataTypeStr=single  SaturationOutMin=[]  SaturationOutMax=[]  PParamDataTypeStr=single  PParamMin=[]  PParamMax=[]  IParamDataTypeStr=single  IParamMin=[]  IParamMax=[]  DParamDataTypeStr=single  DParamMin=[]  DParamMax=[]  NParamMin=[]  NParamMax=[]  KbParamMin=[]  KbParamMax=[]  KtParamMin=[]  KtParamMax=[]  KbOutMin=[]  KbOutMax=[]  KtOutMin=[]  KtOutMax=[]  IntegratorOutDataTypeStr=single  IntegratorOutMin=[]  IntegratorOutMax=[]  FilterOutMin=[]  FilterOutMax=[]  SumI1OutMin=[]  SumI1OutMax=[]  SumI2OutMin=[]  SumI2OutMax=[]  SumI3OutMin=[]  SumI3OutMax=[]  SumI4OutMin=[]  SumI4OutMax=[]  SumDOutMin=[]  SumDOutMax=[]  SumAccumDataTypeStr=single  DifferentiatorOutDataTypeStr=single  DifferentiatorOutMin=[]  DifferentiatorOutMax=[]  FilterDiffOutCoefMin=[]  FilterDiffOutCoefMax=[]  ReciprocalOutMin=[]  ReciprocalOutMax=[]  SumDenOutMin=[]  SumDenOutMax=[]  SumNumOutMin=[]  SumNumOutMax=[]  DivideOutMin=[]  DivideOutMax=[]  IntegratorContinuousStateAttributes=''  IntegratorStateMustResolveToSignalObject=off  IntegratorRTWStateStorageClass=Auto  FilterContinuousStateAttributes=''  FilterStateMustResolveToSignalObject=off  FilterRTWStateStorageClass=Auto  ParallelPVariant=ExternalParameters  IdealPVariant=Disabled  IVariant=ExternalParameters  DVariant=ExternalParameters  IntegratorVariant=Discrete  SatVariant=Enabled  AWVariant=DiscClampingParallel  PCopyVariant=Disabled  TRVariant=Disabled  FdbkBlocksVariant=Feedback  IdealPFdbkVariant=Passthrough  SatFdbkVariant=Passthrough  DerivativeFilterVariant=Differentiator  NVariant=Passthrough  NCopyVariant=Disabled_SignalSpec  FilterICVariant=InternalICsDifferentiator  IntegratorICVariant=InternalICs  ExternalResetVariant=Disabled  TRSumVariant=Passthrough  SumFdbkVariant=Enabled  SumVariant=Sum_PID
  roll_cmd : Outport
  pitch_cmd : Outport  Port=2
  wires:
  roll_control/1 -> roll_cmd/1
  Demux4/3 -> pitch_control/4
  Demux4/2 -> pitch_control/3
  Demux4/1 -> pitch_control/2
  pitch_params/1 -> Demux4/1
  Demux3/3 -> roll_control/4
  Demux3/2 -> roll_control/3
  Demux3/1 -> roll_control/2
  pitch_control/1 -> Gain/1
  e_roll/1 -> roll_control/1
  e_pitch/1 -> pitch_control/1
  roll_params/1 -> Demux3/1
  Gain/1 -> pitch_cmd/1

== matlab function Bixler_w_autopilot_sepTaskRate/MATLAB Function1 ==
  data: u input uint16; y output uint16
function y = invertpwm(u)

y = uint16(1500-(single(u)-1500));

== matlab function Bixler_w_autopilot_sepTaskRate/MATLAB Function ==
  data: u input uint16; y output uint16
function y = invertpwm(u)

y = uint16(1500-(single(u)-1500));

== matlab function Bixler_w_autopilot_sepTaskRate/MATLAB Function2 ==
  data: signals input uint16; y output single
function y = pwm2signal(signals)

y = single(signals);
% Shift to center
y = y-1500;
% Range is ~1000-2000, ie +-500, but in is +-1
y = y./500;

== matlab function Bixler_w_autopilot_sepTaskRate/MATLAB Function3 ==
  data: signals input; y output uint16
function y = signal2pwm(signals)

y = zeros(size(signals)); % y is hard set to uint16


% Range is ~1000-2000, ie +-500, but in is +-1
signals = signals.*500;
% Shift to center PWM
signals = signals+1500;
y = uint16(signals);

== matlab function Bixler_w_autopilot_sepTaskRate/MATLAB Function4 ==
  data: switcher input uint16; pP output single; adjuster input uint16; pI output single; pD output single; enabler input uint16; ControlSelector input uint16; rP output single; rI output single; rD output single
function [pP,pI,pD,rP,rI,rD] = fcn(switcher, adjuster, enabler, ControlSelector)

persistent pkP pkI pkD rkP rkI rkD;
if isempty(pkP)
    pkP = single(1);
end
if isempty(pkI)
    pkI = single(0.4);
end
if isempty(pkD)
    pkD = single(0.025);
end
if isempty(rkP)
    rkP = single(1);
end
if isempty(rkI)
    rkI = single(0.4);
end
if isempty(rkD)
    rkD = single(0.05);
end

if enabler>1500
    if ControlSelector < 1400 % Top, Roll controll
        if switcher < 1400 % Top, P
            rkP = 1+(single(adjuster)-1500)./500; 
        elseif switcher > 1600 % Bottom, D
            rkD = 0.05+0.05*(single(adjuster)-1500)./500;
        else
            rkI = 0.4+0.4*(single(adjuster)-1500)./500;
        end
    elseif ControlSelector < 1600 % Mid, Pitch control
        if switcher < 1400 % Top, P
            pkP = 1+(single(adjuster)-1500)./500; 
        elseif switcher > 1600 % Bottom, D
            pkD = 0.025+0.025*(single(adjuster)-1500)./500;
        else
            pkI = 0.4+0.4*(single(adjuster)-1500)./500;
        end
    else
        % No controller set here yet
    end
end

pP = pkP;
pI = pkI;
pD = pkD;
rP = rkP;
rI = rkI;
rD = rkD;

== matlab function Bixler_w_autopilot_sepTaskRate/ModeSelector ==
  data: selector input uint16; cmds output uint16 size=[2,1]; manual_cmds input uint16; FBW_cmds input uint16; enableFBW output boolean; enableAuto output; auto_cmds input
function [cmds,enableFBW,enableAuto] = fcn(selector, manual_cmds, FBW_cmds, auto_cmds)

if selector>1600 % Auto mode, stick down on remote
    cmds = auto_cmds;
    enableFBW = false;
    enableAuto = true;
elseif selector>1400% Midpoint, as I flew at MUST first time
    cmds = FBW_cmds;
    enableFBW = true;
    enableAuto = false;
else
    cmds = manual_cmds; % As midpoint, but less pitch sensitive.
    enableFBW = false;
    enableAuto = false;
end

== matlab function Bixler_w_autopilot_sepTaskRate/MATLAB Function10 ==
  data: signals input; y output uint16
function y = signal2pwm(signals)

y = zeros(size(signals)); % y is hard set to uint16


% Range is ~1000-2000, ie +-500, but in is +-1
signals = signals.*500;
% Shift to center PWM
signals = signals+1500;
y = uint16(signals);

== matlab function Bixler_w_autopilot_sepTaskRate/linegenerator ==
  settings: updateMethod=DISCRETE
  data: r input single; rspeed output single; wpN output single; dist2wp output single; linevec output single; vec2line output single; wp_r output single; waypoints input single; numwp input single
function [rspeed,wpN, dist2wp, linevec, vec2line, wp_r] = LineGenerator( r, waypoints, numwp)

% Keep track of which waypoint we are going to
persistent waypointno;
persistent wp;
persistent wp_prev;
if isempty(waypointno)
    waypointno=single(2);
    wp=waypoints(waypointno,:)';
    wp_prev=waypoints(waypointno-1,:)';
end

%initialize variables
rspeed = single(0);
vec2line = single([0,0,0])';

% if current waypoint is the start wp/home wp jump immediately to next.
dist2wp = sqrt( sum( (wp(1:2)-r(1:2)).^2 ) ); % We only count horizontal distance!
if dist2wp <= wp(5)
    if waypointno < numwp
        waypointno = waypointno+1;
    else
        waypointno = single(1); % 
    end
    wp_prev = wp;
    wp = waypoints(waypointno,:)';
end
rspeed = wp(4);
wp_r = wp(1:3); % Next waypoint position, v has been scaled away thus wp_r

% find vector between last waypoint and current target
linevec = (wp(1:3)-wp_prev(1:3))./sqrt( sum((wp(1:3)-wp_prev(1:3)).^2) );

if  dot(linevec, wp(1:3)-r) < 0 
    linevec(1:3)=-linevec(1:3);
end

a = wp_prev(1:3);               % Points to "start of line"
n = linevec;                    % Points toward next wp
vec2line = a-r - dot(a-r,n)*n;  % Points toward closest point on line
wpN = waypointno;
